simulink model "RLCCircuit_SIM"  (R2012b)
settings: Solver=ode3  StartTime=0.0  StopTime=10.0  FixedStep=0.001  RelTol=1e-3
values from neighbouring files (symbols this model uses):
  C = 0.0001    [RLCCircuit.m]
  L = 1    [RLCCircuit.m]
  R = 100    [RLCCircuit.m]
  V = 10    [RLCCircuit.m]
settings Model: Creator=aluno  LastModifiedBy=aluno

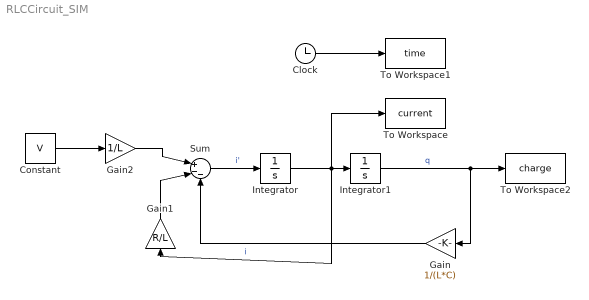
== system RLCCircuit_SIM ==
  Clock : Clock
  Constant : Constant  Value=V
  Gain : Gain  Gain=1/(L*C)
  Gain1 : Gain  Gain=R/L
  Gain2 : Gain  Gain=1/L
  Integrator : Integrator
  Integrator1 : Integrator
  Sum : Sum  Inputs=|+--
  To Workspace : ToWorkspace  VariableName=current  SampleTime=-1
  To Workspace1 : ToWorkspace  VariableName=time  SampleTime=-1
  To Workspace2 : ToWorkspace  VariableName=charge  SampleTime=-1
  wires:
  Integrator/1 -> To Workspace/1, Gain1/1, Integrator1/1  "i"
  Integrator1/1 -> To Workspace2/1, Gain/1  "q"
  Sum/1 -> Integrator/1  "i'"
  Gain/1 -> Sum/3
  Gain1/1 -> Sum/2
  Gain2/1 -> Sum/1
  Constant/1 -> Gain2/1
  Clock/1 -> To Workspace1/1
